simulink model "selector_port_matrix_test"  (Simulink 8.4)
settings: Solver=VariableStepDiscrete  StartTime=0.0  StopTime=0  MaxStep=1  RelTol=1e-3
settings Model: Creator=arnaud  LastModifiedBy=arnaud
settings DataIOCC: ExternalInput=xin  SaveFormat=Structure

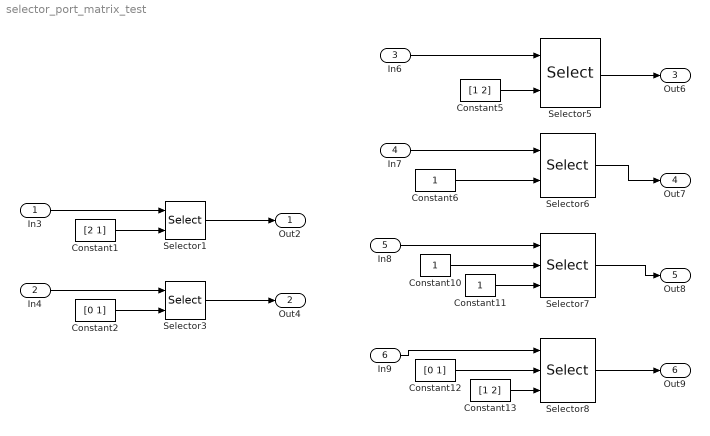
== system selector_port_matrix_test ==
  In3 : Inport  PortDimensions=[2 3]
  In4 : Inport  Port=2  PortDimensions=[2 3]
  In6 : Inport  Port=3  PortDimensions=3
  In7 : Inport  Port=4  PortDimensions=[2 3]
  In8 : Inport  Port=5  PortDimensions=[2 3]
  In9 : Inport  Port=6  PortDimensions=[2 3]
  Constant1 : Constant  Value=[2 1]
  Constant10 : Constant
  Constant11 : Constant
  Constant12 : Constant  Value=[0 1]
  Constant13 : Constant  Value=[1 2]
  Constant2 : Constant  Value=[0 1]
  Constant5 : Constant  Value=[1 2]
  Constant6 : Constant
  Selector1 : Selector  NumberOfDimensions=2  InputPortWidth=3  IndexOptions=Index vector (port),Index vector (dialog)  Indices=[2 1],1  OutputSizes=1,2
  Selector3 : Selector  NumberOfDimensions=2  IndexMode=Zero-based  InputPortWidth=3  IndexOptions=Index vector (port),Index vector (dialog)  Indices=[1 0],1  OutputSizes=1,2
  Selector5 : Selector  NumberOfDimensions=2  InputPortWidth=3  IndexOptions=Select all,Index vector (port)  Indices=[2 1],1  OutputSizes=1,2
  Selector6 : Selector  NumberOfDimensions=2  IndexMode=Zero-based  InputPortWidth=3  IndexOptions=Index vector (port),Select all  Indices=[1 0],1  OutputSizes=1,2
  Selector7 : Selector  NumberOfDimensions=2  InputPortWidth=3  IndexOptions=Index vector (port),Index vector (port)  Indices=0,1  OutputSizes=1,2
  Selector8 : Selector  NumberOfDimensions=2  IndexMode=Zero-based  InputPortWidth=3  IndexOptions=Index vector (port),Index vector (port)  Indices=0,1  OutputSizes=1,2
  Out2 : Outport
  Out4 : Outport  Port=2
  Out6 : Outport  Port=3
  Out7 : Outport  Port=4
  Out8 : Outport  Port=5
  Out9 : Outport  Port=6
  wires:
  Selector1/1 -> Out2/1
  In3/1 -> Selector1/1
  Selector3/1 -> Out4/1
  In4/1 -> Selector3/1
  Constant1/1 -> Selector1/2
  Constant2/1 -> Selector3/2
  Selector5/1 -> Out6/1
  In6/1 -> Selector5/1
  Selector6/1 -> Out7/1
  In7/1 -> Selector6/1
  Selector7/1 -> Out8/1
  In8/1 -> Selector7/1
  Constant10/1 -> Selector7/2
  Constant5/1 -> Selector5/2
  Constant6/1 -> Selector6/2
  Constant11/1 -> Selector7/3
  Selector8/1 -> Out9/1
  In9/1 -> Selector8/1
  Constant12/1 -> Selector8/2
  Constant13/1 -> Selector8/3
